simulink model "satellite_sim"  (R2016b)
settings: Solver=ode45  StartTime=0.0  StopTime=300  RelTol=1e-3  EnableMultiTasking=on
InitFcn:
  | addpath ./..
  | satelliteParam
  | satelliteParamHW8
undefined symbols (not defined in the file or in its folder): P, satellite_animation
settings Model: Creator=beard  LastModifiedBy=mclain
settings DataIOCC: LimitDataPoints=on  SaveFormat=Array  SignalLoggingSaveFormat=ModelDataLogs
settings OptimizationCC: ExpressionDepthLimit=2147483647  InitFltsAndDblsToZero=on  LifeSpan=inf
settings DebuggingCC: UnderspecifiedInitializationDetection=Classic  MergeDetectMultiDrivingBlocksExec=none  SolverPrmCheckMsg=warning  FcnCallInpInsideContextMsg=warning  StateNameClashWarn=warning  SFUnexpectedBacktrackingDiag=warning  SFNoUnconditionalDefaultTransitionDiag=warning  SFExecutionAtInitializationDiag=none
settings HardwareCC: ProdBitPerPointer=32  ProdBitPerSizeT=32  ProdBitPerPtrDiffT=32  ProdLargestAtomicFloat=None  ProdIntDivRoundTo=Undefined  ProdEndianess=Unspecified  ProdWordSize=32  ProdHWDeviceType=32-bit Generic
settings ModelReferenceCC: PropagateSignalLabelsOutOfModel=off
settings GRTTargetCC: TargetLangStandard=C89/C90 (ANSI)  GeneratePreprocessorConditionals=Disable all  CombineOutputUpdateFcns=off  GRTInterface=on
settings ConfigComp: CovMetricSettings=dw  CovHtmlReporting=on  CovSaveCumulativeToWorkspaceVar=on  CovSaveSingleToWorkspaceVar=on  CovExternalEMLEnable=off

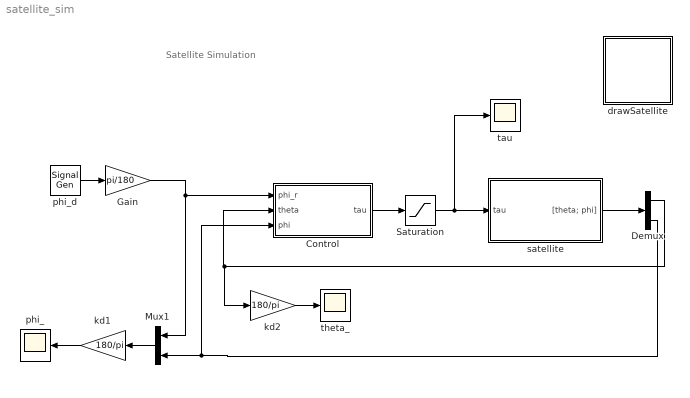
== system satellite_sim ==
  note: Satellite Simulation
  Control : Subsystem
  Demux : Demux  Outputs=2
  Gain : Gain  Gain=pi/180
  Mux1 : Mux  Inputs=2
  Saturation : Saturate  UpperLimit=P.taumax  LowerLimit=-P.taumax
  drawSatellite : Subsystem
      mask Display: image(imread('tv.jpg'))
  kd1 : Gain  Gain=180/pi
  kd2 : Gain  Gain=180/pi
  phi_ : Scope
  phi_d : SignalGenerator  WaveForm=square  Amplitude=15  Frequency=.015
  satellite : Subsystem
  tau : Scope
  theta_ : Scope
  wires:
  satellite/1("[theta; phi]") -> Demux/1
  phi_d/1 -> Gain/1
  Saturation/1 -> satellite/1(tau), tau/1
  Demux/1 -> kd2/1, Control/2(theta)
  Control/1(tau) -> Saturation/1
  Mux1/1 -> kd1/1
  kd1/1 -> phi_/1
  Demux/2 -> Mux1/2, Control/3(phi)
  Gain/1 -> Mux1/1, Control/1(phi_r)
  kd2/1 -> theta_/1

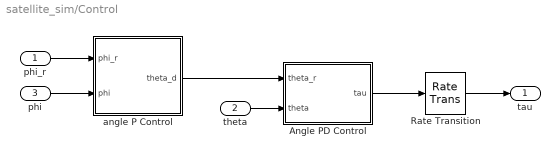
== system satellite_sim/Control ==
  phi_r : Inport
  theta : Inport  Port=2
  phi : Inport  Port=3
  "Angle PD Control " : Subsystem
  Rate Transition : RateTransition  OutPortSampleTime=P.Ts
  angle P Control : Subsystem
  tau : Outport
  wires:
  phi/1 -> angle P Control/2(phi)
  angle P Control/1(theta_d) -> "Angle PD Control "/1(theta_r)
  theta/1 -> "Angle PD Control "/2(theta)
  phi_r/1 -> angle P Control/1(phi_r)
  "Angle PD Control "/1(tau) -> Rate Transition/1
  Rate Transition/1 -> tau/1

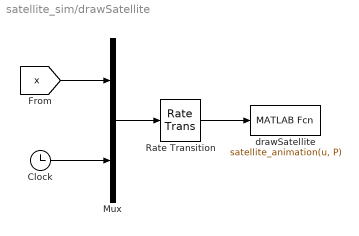
== system satellite_sim/drawSatellite ==
  Clock : Clock
  Mux : Mux  Inputs=2
  Rate Transition : RateTransition  OutPortSampleTime=P.t_plot
  drawSatellite : MATLABFcn  MATLABFcn=satellite_animation(u, P)  OutputDimensions=0
  wires:
  Rate Transition/1 -> drawSatellite/1
  Clock/1 -> Mux/2
  [x] -> Mux/1
  Mux/1 -> Rate Transition/1

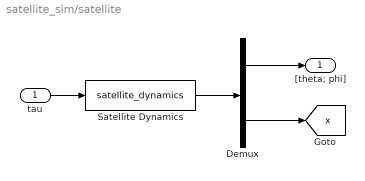
== system satellite_sim/satellite ==
  tau : Inport
  Demux : Demux  Outputs=[2;4]
  Satellite Dynamics : S-Function  FunctionName=satellite_dynamics  Parameters=P  SFunctionDeploymentMode=off  EnableBusSupport=off
  "[theta; phi]" : Outport
  tag scope: x=global
  wires:
  tau/1 -> Satellite Dynamics/1
  Satellite Dynamics/1 -> Demux/1
  Demux/1 -> "[theta; phi]"/1
  Demux/2 -> [x]

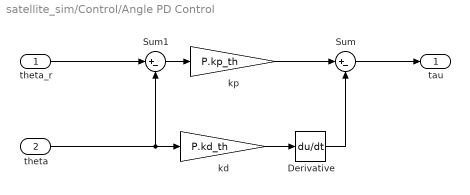
== system satellite_sim/Control/Angle PD Control  ==
  theta_r : Inport
  theta : Inport  Port=2
  Derivative : Derivative
  Sum : Sum  Inputs=|+-
  Sum1 : Sum  Inputs=|+-
  kd : Gain  Gain=P.kd_th
  kp : Gain  Gain=P.kp_th
  tau : Outport
  wires:
  Derivative/1 -> Sum/2
  kd/1 -> Derivative/1
  kp/1 -> Sum/1
  Sum1/1 -> kp/1
  theta/1 -> Sum1/2, kd/1
  Sum/1 -> tau/1
  theta_r/1 -> Sum1/1

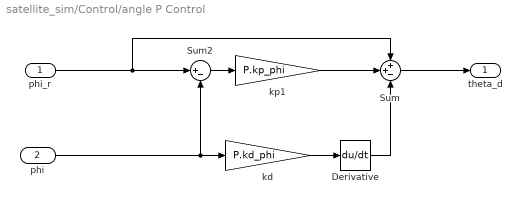
== system satellite_sim/Control/angle P Control ==
  phi_r : Inport
  phi : Inport  Port=2
  Derivative : Derivative
  Sum : Sum  Inputs=++-
  Sum2 : Sum  Inputs=|+-
  kd : Gain  Gain=P.kd_phi
  kp1 : Gain  Gain=P.kp_phi
  theta_d : Outport
  wires:
  kd/1 -> Derivative/1
  Sum2/1 -> kp1/1
  phi/1 -> Sum2/2, kd/1
  Sum/1 -> theta_d/1
  phi_r/1 -> Sum2/1, Sum/1
  Derivative/1 -> Sum/3
  kp1/1 -> Sum/2
